simulink library "BeagleBoneBlackCom"  (R2014b)
settings: Solver=ode45  StartTime=0.0  StopTime=10.0  RelTol=1e-3
settings Model: Creator=Sebastian  LastModifiedBy=Sebastian

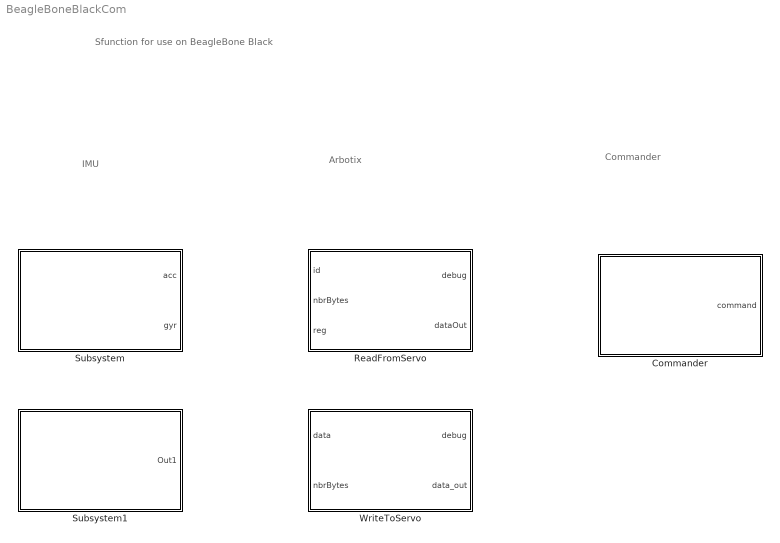
== system BeagleBoneBlackCom ==
  note: Sfunction for use on BeagleBone Black
  note: Commander
  note: IMU
  note: Arbotix
  Commander : Subsystem  mask{portNbr=Uart 2}
      mask help:
      | This function reads the next available message from the commander.
      | Message are sent at a rate of 30 Hz from the commander.
      mask TypeOptions portNbr: Uart 1 | Uart 2 | Uart 4 | Uart 5
      mask Display:
      | gr_opt = get_param(gcb, 'portNbr');
      | fprintf('Commander\n\n\n')
      | fprintf('%s',gr_opt)
      | %port_label('output',1,'data')
      | port_label('output',1,'command')
      | %port_label('output',3,'debug')
  ReadFromServo : Subsystem
  Subsystem : Subsystem  mask(MPU-9150){accSens=2 g, gyroSens=1000 degree/s}
      mask prompts: accSens "Accelerometer"; gyroSens "Gyro"
      mask help: Sampletime is fixed to 100 Hz.
      mask TypeOptions accSens: 2 g | 4 g | 8 g | 16 g
      mask TypeOptions gyroSens: 250 degree/s | 500 degree/s | 1000 degree/s | 2000 degree/s
      mask Display:
      | fprintf('MPU-9150\n\n\n')
      | fprintf('Accelerometer %d g',2^accSens)
      | fprintf('\n\n\n Gyro %d degree/sec',2^(gyroSens-1)*250)
      | port_label('output',1,'acc')
      | port_label('output',2,'gyro')
  Subsystem1 : Subsystem
      mask Display:
      | fprintf('MPU-9150\n\n\n')
      | fprintf('Sensor fusion')
      | fprintf('\n\n\nEuler angles')
      | port_label('output',1,'angles')
  WriteToServo : Subsystem

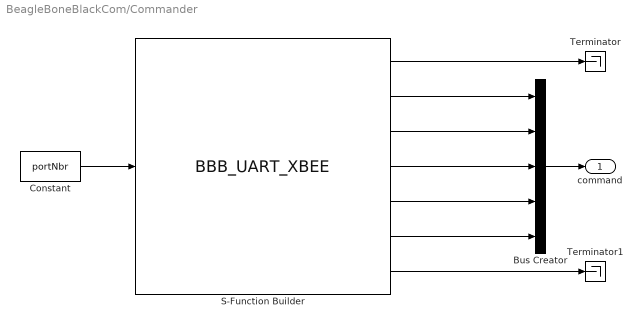
== system BeagleBoneBlackCom/Commander ==
  Bus Creator : BusCreator  Inputs=5  OutDataTypeStr=Bus: Command
      settings: InheritFromInputs=off
  Constant : Constant  Value=portNbr  OutDataTypeStr=int8  SampleTime=0.0125
      settings: AttributesFormatString=Sample time = %<SampleTime>
  S-Function Builder : S-Function  InitFcn=try, set_param(gcb,'FunctionName','BBB_UART_XBEE'), end  FunctionName=BBB_UART_XBEE  SFunctionModules=BBB_UART_XBEE_wrapper  EnableBusSupport=off  mask(S-Function Builder){}
      mask help: Simulink:masks:SFunctionBuilder_MD
      mask init:
      | val = [[.9  0.75 0.75 1 1 .9 .9 1]',[1 1 0.75 0.75 .9 .9 1 .9]'];try , sys = get_param(gcb,'SfunBuilderFcnName');if isempty(sys), sys = get_param(gcb,'FunctionName'); end,catch, sys = get_param(gcb,'FunctionName'); end
      settings: CopyFcn=set_param(gcbh,'LinkStatus','none')  PreSaveFcn=try, set_param(gcb,'FunctionName','BBB_UART_XBEE'), end  OpenFcn=sfunctionwizard(gcbh)
      mask Display: plot(val(:,1),val(:,2)),disp(sys), port_label('input',1,'portNbr'), port_label('output',1,'data'), port_label('output',2,'walkV'), port_label('output',3,'walkH'), port_label('output',4,'lookV'), port_label('output',5,'lookH'), port_label('output',6,'buttons'), port_label('output',7,'debug')
  Terminator : Terminator
  Terminator1 : Terminator
  command : Outport  OutDataTypeStr=Bus: Command
  wires:
  Constant/1 -> S-Function Builder/1
  S-Function Builder/7 -> Terminator1/1
  S-Function Builder/1 -> Terminator/1
  S-Function Builder/2 -> Bus Creator/1
  S-Function Builder/3 -> Bus Creator/2
  S-Function Builder/4 -> Bus Creator/3
  S-Function Builder/5 -> Bus Creator/4
  S-Function Builder/6 -> Bus Creator/5
  Bus Creator/1 -> command/1

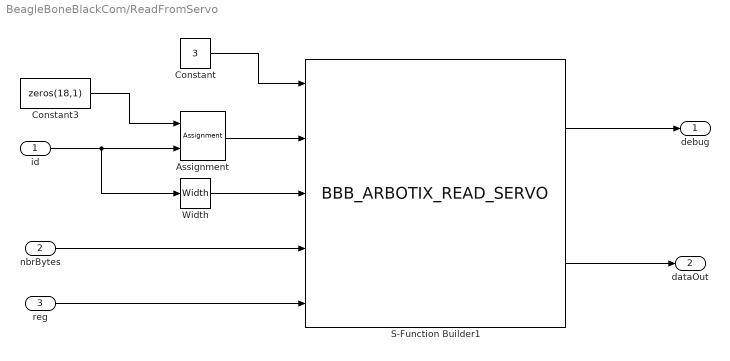
== system BeagleBoneBlackCom/ReadFromServo ==
  id : Inport
  nbrBytes : Inport  Port=2
  reg : Inport  Port=3
  Assignment : Assignment  IndexMode=Zero-based  DiagnosticForDimensions=Warning  IndexOptions=Starting index (dialog)  Indices=0
  Constant : Constant  Value=3  OutDataTypeStr=uint8  SampleTime=-1
      settings: AttributesFormatString=Sample time = %<SampleTime>
  Constant3 : Constant  Value=zeros(18,1)  OutDataTypeStr=uint8  SampleTime=-1
      settings: AttributesFormatString=Sample time = %<SampleTime>
  S-Function Builder1 : S-Function  InitFcn=try, set_param(gcb,'FunctionName','BBB_ARBOTIX_READ_SERVO'), end  FunctionName=BBB_ARBOTIX_READ_SERVO  SFunctionModules=BBB_ARBOTIX_READ_SERVO_wrapper  EnableBusSupport=off  mask(S-Function Builder){}
      mask help: Simulink:masks:SFunctionBuilder_MD
      mask init: same as BeagleBoneBlackCom/Commander/S-Function Builder
      settings: CopyFcn=set_param(gcbh,'LinkStatus','none')  PreSaveFcn=try, set_param(gcb,'FunctionName','BBB_ARBOTIX_READ_SERVO'), end  OpenFcn=sfunctionwizard(gcbh)
      mask Display: plot(val(:,1),val(:,2)),disp(sys), port_label('input',1,'portNbr'), port_label('input',2,'id'), port_label('input',3,'nbrOfServo'), port_label('input',4,'nbrBytes'), port_label('input',5,'reg'), port_label('output',1,'debug'), port_label('output',2,'dataOut')
  Width : Width  DataType=uint8
  debug : Outport
  dataOut : Outport  Port=2
  wires:
  Constant3/1 -> Assignment/1
  Assignment/1 -> S-Function Builder1/2
  S-Function Builder1/1 -> debug/1
  nbrBytes/1 -> S-Function Builder1/4
  Width/1 -> S-Function Builder1/3
  Constant/1 -> S-Function Builder1/1
  S-Function Builder1/2 -> dataOut/1
  id/1 -> Width/1, Assignment/2
  reg/1 -> S-Function Builder1/5

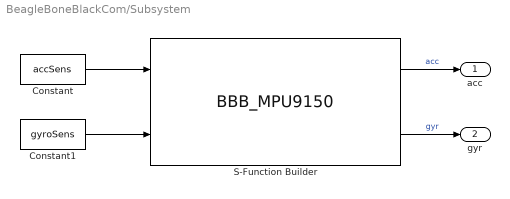
== system BeagleBoneBlackCom/Subsystem ==
  Constant : Constant  Value=accSens  OutDataTypeStr=int8  SampleTime=0.01
      settings: AttributesFormatString=Sample time = %<SampleTime>
  Constant1 : Constant  Value=gyroSens  OutDataTypeStr=int8  SampleTime=0.01
      settings: AttributesFormatString=Sample time = %<SampleTime>
  S-Function Builder : S-Function  InitFcn=try, set_param(gcb,'FunctionName','BBB_MPU9150'), end  FunctionName=BBB_MPU9150  SFunctionModules=BBB_MPU9150_wrapper  EnableBusSupport=off  mask(S-Function Builder){}
      mask help: Simulink:masks:SFunctionBuilder_MD
      mask init: same as BeagleBoneBlackCom/Commander/S-Function Builder
      settings: CopyFcn=set_param(gcbh,'LinkStatus','none')  PreSaveFcn=try, set_param(gcb,'FunctionName','BBB_MPU9150'), end  OpenFcn=sfunctionwizard(gcbh)
      mask Display: plot(val(:,1),val(:,2)),disp(sys), port_label('input',1,'accSens'), port_label('input',2,'gyroSens'), port_label('output',1,'acc'), port_label('output',2,'gyr')
  acc : Outport
  gyr : Outport  Port=2
  wires:
  S-Function Builder/2 -> gyr/1  "gyr"
  S-Function Builder/1 -> acc/1  "acc"
  Constant/1 -> S-Function Builder/1
  Constant1/1 -> S-Function Builder/2

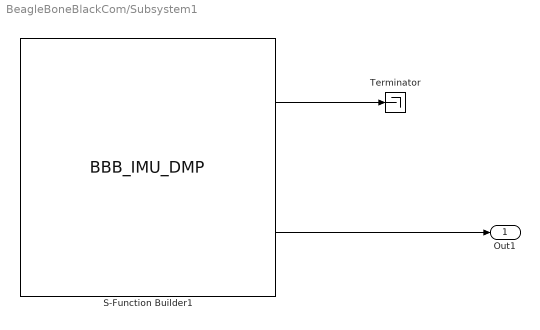
== system BeagleBoneBlackCom/Subsystem1 ==
  S-Function Builder1 : S-Function  InitFcn=try, set_param(gcb,'FunctionName','BBB_IMU_DMP'), end  FunctionName=BBB_IMU_DMP  Parameters=int16([-17524,17966,-17130,17078,-18186,18790]),int16([-250,134,-161,289,-145,236])  SFunctionModules=BBB_IMU_DMP_wrapper  EnableBusSupport=off  mask(S-Function Builder){}
      mask help: Simulink:masks:SFunctionBuilder_MD
      mask init: same as BeagleBoneBlackCom/Commander/S-Function Builder
      settings: CopyFcn=set_param(gcbh,'LinkStatus','none')  PreSaveFcn=try, set_param(gcb,'FunctionName','BBB_IMU_DMP'), end  OpenFcn=sfunctionwizard(gcbh)
      mask Display: plot(val(:,1),val(:,2)),disp(sys), port_label('output',1,'debug'), port_label('output',2,'angle')
  Terminator : Terminator
  Out1 : Outport
  wires:
  S-Function Builder1/2 -> Out1/1
  S-Function Builder1/1 -> Terminator/1

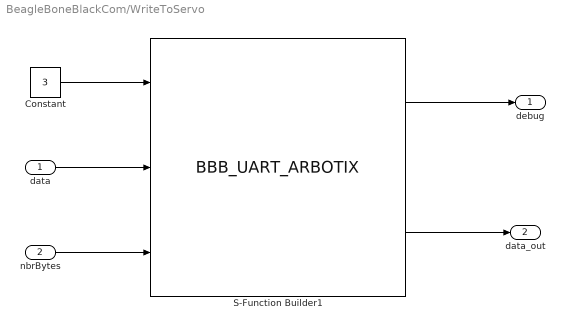
== system BeagleBoneBlackCom/WriteToServo ==
  data : Inport
  nbrBytes : Inport  Port=2
  Constant : Constant  Value=3  OutDataTypeStr=uint8  SampleTime=-1
      settings: AttributesFormatString=Sample time = %<SampleTime>
  S-Function Builder1 : S-Function  InitFcn=try, set_param(gcb,'FunctionName','BBB_UART_ARBOTIX'), end  FunctionName=BBB_UART_ARBOTIX  SFunctionModules=BBB_UART_ARBOTIX_wrapper  EnableBusSupport=off  mask(S-Function Builder){}
      mask help: Simulink:masks:SFunctionBuilder_MD
      mask init: same as BeagleBoneBlackCom/Commander/S-Function Builder
      settings: CopyFcn=set_param(gcbh,'LinkStatus','none')  PreSaveFcn=try, set_param(gcb,'FunctionName','BBB_UART_ARBOTIX'), end  OpenFcn=sfunctionwizard(gcbh)
      mask Display: plot(val(:,1),val(:,2)),disp(sys), port_label('input',1,'portNbr'), port_label('input',2,'data'), port_label('input',3,'nbrBytes'), port_label('output',1,'debug'), port_label('output',2,'data_out')
  debug : Outport
  data_out : Outport  Port=2
  wires:
  S-Function Builder1/1 -> debug/1
  nbrBytes/1 -> S-Function Builder1/3
  data/1 -> S-Function Builder1/2
  Constant/1 -> S-Function Builder1/1
  S-Function Builder1/2 -> data_out/1
